simulink model "controller_testing_OPEN_LOOP"  (R2023b)
settings: Solver=FixedStepAuto  StartTime=0.0  StopTime=3180  FixedStep=0.015  RelTol=1e-3
undefined symbols (not defined in the file): tvs
libraries: dspstat3 x4
settings Model: SimulationMode=rapid-accelerator  Creator=Inver  LastModifiedBy=Inver
settings DataIOCC: ExternalInput=x2023_5_11_controller_testing_RA.getElement('throttle'),x2023_5_11_controller_testing_RA.getElement('steering_angle'),x2023_5_11_controller_testing_RA.getElement('pack_voltage'),x2023_5_11_controller_testing_RA.getElement('left_wheel_omega_filt'),x2023_5_11_controller_testing_RA.getElement('gps_vel_n_filt'),x2023_5_11_controller_testing_RA.getElement('pack_current'),x2023_5_11_controller_testing_RA.getElement('left_temp_motor'),x2023_5_11_controller_testing_RA.getElement('left_temp_controller'),x2023_5_11_controller_testing_RA.getElement('imu_accel_x'),x2023_5_11_controller_testing_RA.getElement('right_wheel_omega_filt'),x2023_5_11_controller_testing_RA.getElement('gps_vel_e_filt'),x2023_5_11_controller_testing_RA.getElement('gps_vel_d_filt'),x2023_5_11_controller_testing_RA.getElement('imu_gyro_x'),x2023_5_11_controller_testing_RA.getElement('imu_gyro_y'),x2023_5_11_controller_testing_RA.getElement('imu_gyro_z'),x2023_5_11_controller_testing_RA.getElement('right_temp_motor'),x2023_5_11_controller_testing_RA.getElement('right_temp_controller'),x2023_5_11_controller_testing_RA.getElement('imu_accel_y'),x2023_5_11_controller_testing_RA.getElement('imu_accel_z')  LoadExternalInput=on
settings OptimizationCC: DefaultParameterBehavior=Inlined  UseDivisionForNetSlopeComputation=on  GainParamInheritBuiltInType=on  UseFloatMulNetSlope=on  UseSpecifiedMinMax=on  InlineInvariantSignals=on  PassReuseOutputArgsAs=Individual arguments  ZeroExternalMemoryAtStartup=off  ZeroInternalMemoryAtStartup=off  NoFixptDivByZeroProtection=on  EfficientFloat2IntCast=on  LifeSpan=1  OptimizeBlockOrder=speed  DifferentSizesBufferReuse=on  OptimizationPriority=Speed  MultiThreadedLoops=on  EfficientTunableParamExpr=on
settings DebuggingCC: ReadBeforeWriteMsg=DisableAll  WriteAfterWriteMsg=DisableAll  WriteAfterReadMsg=DisableAll  MultiTaskDSMMsg=none  ParameterTunabilityLossMsg=error
settings HardwareCC: ProdBitPerPointer=32  ProdBitPerSizeT=32  ProdBitPerPtrDiffT=32  ProdLargestAtomicInteger=Long  ProdLargestAtomicFloat=Double  ProdWordSize=32  ProdLongLongMode=on  ProdHWDeviceType=ARM Compatible->ARM Cortex-M
settings SFSimCC: SimCustomHeaderCode="#include \"simplex.h\""  SimUserSources=simplex.c  SFSimEcho=off  MATLABDynamicMemAlloc=off
settings RTWCC: Description=Embedded Coder  SystemTargetFile=ert.tlc  GenCodeOnly=on  PackageGeneratedCodeAndArtifacts=on  TemplateMakefile=ert_default_tmf  Toolchain=GNU Tools for ARM Embedded Processors  BuildConfiguration=Faster Runs
settings CodeAppCC: ForceParamTrailComments=on  IgnoreCustomStorageClasses=off  OperatorAnnotations=on  SimulinkDataObjDesc=on  SFDataObjDesc=on  CustomSymbolStrGlobalVar=rt$N$M  CustomSymbolStrType=$N$M  CustomSymbolStrFcn=$N$M$F  CustomSymbolStrMacro=$N$M  InsertBlockDesc=on
settings ERTTargetCC: TargetLangStandard=C99 (ISO)  GenerateSampleERTMain=on  IncludeMdlTerminateFcn=off  CombineSignalStateStructs=on  SupportAbsoluteTime=off  CodeInterfacePackaging=Reusable function  SupportComplex=off  SupportNonInlinedSFcns=on  InlinedParameterPlacement=NonHierarchical  RootIOFormat=Structure reference  ERTCustomFileTemplate=example_file_process.tlc  GlobalDataDefinition=InSeparateSourceFile  DataDefinitionFile=data.c  GlobalDataReference=InSeparateHeaderFile  ERTFilePackagingFormat=CompactWithDataFile  DataReferenceFile=data.h  EnableUserReplacementTypes=on

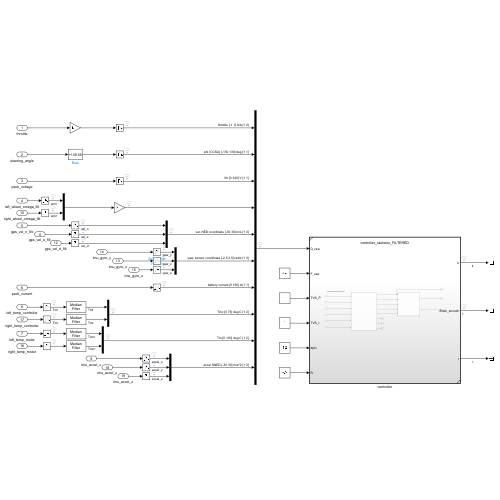
[thumbnail: Simulink's stored preview of the top-level diagram]
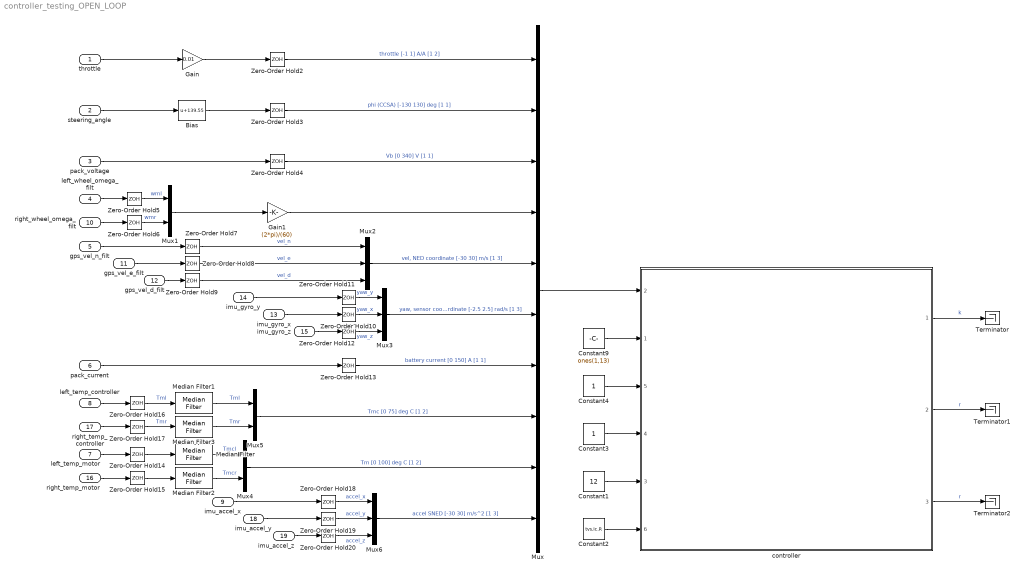
== system controller_testing_OPEN_LOOP ==
  throttle : Inport
  steering_angle : Inport  Port=2
  pack_voltage : Inport  Port=3
  left_wheel_omega_filt : Inport  Port=4
  gps_vel_n_filt : Inport  Port=5
  pack_current : Inport  Port=6
  left_temp_motor : Inport  Port=7
  left_temp_controller : Inport  Port=8
  imu_accel_x : Inport  Port=9
  right_wheel_omega_filt : Inport  Port=10
  gps_vel_e_filt : Inport  Port=11
  gps_vel_d_filt : Inport  Port=12
  imu_gyro_x : Inport  Port=13
  imu_gyro_y : Inport  Port=14
  imu_gyro_z : Inport  Port=15
  right_temp_motor : Inport  Port=16
  right_temp_controller : Inport  Port=17
  imu_accel_y : Inport  Port=18
  imu_accel_z : Inport  Port=19
  Bias : Bias  Bias=139.55  SaturateOnIntegerOverflow=off
  Constant1 : Constant  Value=12
  Constant2 : Constant  Value=tvs.ic.R
  Constant3 : Constant
  Constant4 : Constant
  Constant9 : Constant  Value=ones(1,13)  OutDataTypeStr=boolean
  Gain : Gain  Gain=0.01
  Gain1 : Gain  Gain=(2*pi)/(60)
  Median Filter{,1..3} (4 alike) : dspstat3/Median Filter  WindowLength=150  SimulateUsing=Interpreted execution
      settings: LibrarySourceBlock=|
      | dspfdesign/Median
      | Filter
  Mux : Mux  Inputs=10
  Mux1 : Mux  Inputs=2
  Mux2 : Mux  Inputs=3
  Mux3 : Mux  Inputs=3
  Mux4 : Mux  Inputs=2
  Mux5 : Mux  Inputs=2
  Mux6 : Mux  Inputs=3
  Terminator : Terminator
  Terminator1 : Terminator
  Terminator2 : Terminator
  Zero-Order Hold{2..20} (19 alike) : ZeroOrderHold  SampleTime=tvs.const.ts
  controller : Subsystem  TreatAsAtomicUnit=on  SystemSampleTime=tvs.const.ts  ReferencedSubsystem=controller_skeleton_FILTERED
      settings: PortSchema="{\"entries\":[{\"content\":{\"sides\":[{\"content\":{\"connectorIds\":[\"In2\",\"In1\",\"In5\",\"In4\",\"In3\",\"In6\"]},\"type\":\"ConnectorPlacement.EquallySpacedRectSide\",\"uuid\":\"52b1df42-6e7f-45d3-b7c9-232c4418f487\"},{\"content\":{\"connectorIds\":[\"Out1\",\"Out2\",\"Out3\"],\"side\":\"RIGHT\"},\"type\":\"ConnectorPlacement.EquallySpacedRectSide\",\"uuid\":\"e4c52b5d-e43f-4131-af39-863e21bd5493\"},{\"content\":{\"side\":\"TOP\"},\"type\":\"ConnectorPlacement.EquallySpacedRectSide\",\"uuid\":\"e8efffec-e2c6-4a68-bbcf-545da82a33a9\"}]},\"type\":\"ConnectorPlacement.EquallySpacedConnector\",\"uuid\":\"e642afc6-31fe-4ac7-95bb-2149c1d24da1\"}],\"packageUris\":[\"http://schema.mathworks.com/mf0/Connector/R2020b\"],\"version\":\"1.0\"}"
  wires:
  controller/1 -> Terminator/1  "k"
  throttle/1 -> Gain/1
  steering_angle/1 -> Bias/1
  controller/3 -> Terminator2/1  "r"
  pack_voltage/1 -> Zero-Order Hold4/1
  pack_current/1 -> Zero-Order Hold13/1
  controller/2 -> Terminator1/1  "r"
  gps_vel_n_filt/1 -> Zero-Order Hold7/1
  Mux3/1 -> Mux/6  "yaw, sensor coordinate [-2.5 2.5] rad/s [1 3]"
  left_wheel_omega_filt/1 -> Zero-Order Hold5/1
  Constant1/1 -> controller/3
  Constant3/1 -> controller/4
  Constant4/1 -> controller/5
  Constant9/1 -> controller/1
  Mux/1 -> controller/2
  Mux6/1 -> Mux/10  "accel SNED [-30 30] m/s^2 [1 3]"
  right_wheel_omega_filt/1 -> Zero-Order Hold6/1
  Mux1/1 -> Gain1/1
  gps_vel_d_filt/1 -> Zero-Order Hold9/1
  gps_vel_e_filt/1 -> Zero-Order Hold8/1
  imu_gyro_x/1 -> Zero-Order Hold10/1
  imu_gyro_y/1 -> Zero-Order Hold11/1
  imu_gyro_z/1 -> Zero-Order Hold12/1
  left_temp_motor/1 -> Zero-Order Hold14/1
  right_temp_motor/1 -> Zero-Order Hold15/1
  left_temp_controller/1 -> Zero-Order Hold16/1
  right_temp_controller/1 -> Zero-Order Hold17/1
  imu_accel_x/1 -> Zero-Order Hold18/1
  imu_accel_y/1 -> Zero-Order Hold19/1
  imu_accel_z/1 -> Zero-Order Hold20/1
  Zero-Order Hold2/1 -> Mux/1  "throttle [-1 1] A/A [1 2]"
  Zero-Order Hold3/1 -> Mux/2  "phi (CCSA) [-130 130] deg [1 1]"
  Zero-Order Hold4/1 -> Mux/3  "Vb [0 340] V [1 1]"
  Zero-Order Hold5/1 -> Mux1/1  "wml"
  Zero-Order Hold6/1 -> Mux1/2  "wmr"
  Zero-Order Hold7/1 -> Mux2/1  "vel_n"
  Zero-Order Hold8/1 -> Mux2/2  "vel_e"
  Zero-Order Hold9/1 -> Mux2/3  "vel_d"
  Zero-Order Hold10/1 -> Mux3/2  "yaw_x"
  Zero-Order Hold11/1 -> Mux3/1  "yaw_y"
  Zero-Order Hold12/1 -> Mux3/3  "yaw_z"
  Zero-Order Hold13/1 -> Mux/7  "battery current [0 150] A [1 1]"
  Zero-Order Hold14/1 -> Median Filter/1
  Zero-Order Hold15/1 -> Median Filter2/1
  Zero-Order Hold16/1 -> Median Filter1/1  "Tml"
  Zero-Order Hold17/1 -> Median Filter3/1  "Tmr"
  Zero-Order Hold18/1 -> Mux6/1  "accel_x"
  Zero-Order Hold19/1 -> Mux6/2  "accel_y"
  Zero-Order Hold20/1 -> Mux6/3  "accel_z"
  Gain/1 -> Zero-Order Hold2/1
  Bias/1 -> Zero-Order Hold3/1
  Constant2/1 -> controller/6
  Mux5/1 -> Mux/8  "Tmc [0 75] deg C [1 2]"
  Mux2/1 -> Mux/5  "vel, NED coordinate [-30 30] m/s [1 3]"
  Median Filter/1 -> Mux4/1  "Tmcl"
  Median Filter2/1 -> Mux4/2  "Tmcr"
  Mux4/1 -> Mux/9  "Tm [0 100] deg C [1 2]"
  Median Filter1/1 -> Mux5/1  "Tml"
  Median Filter3/1 -> Mux5/2  "Tmr"
  Gain1/1 -> Mux/4
